simulink model "Model_3"  (R2025b)
settings: Solver=VariableStepAuto  StartTime=0.0  StopTime=10.0  RelTol=1e-3
settings Model: Creator=danielborkovec  LastModifiedBy=danielborkovec

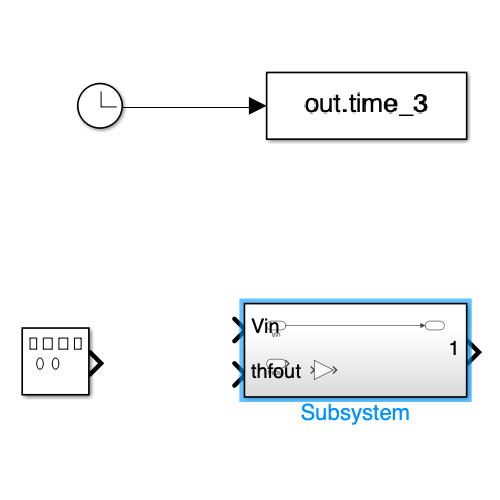
[thumbnail: Simulink's stored preview of the top-level diagram]
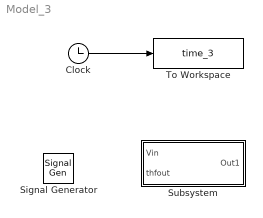
== system Model_3 ==
  Clock : Clock
  Signal Generator : SignalGenerator  Units=rad/sec
  Subsystem : Subsystem
  To Workspace : ToWorkspace  VariableName=time_3  SaveFormat=Timeseries  SampleTime=-1
  wires:
  Clock/1 -> To Workspace/1

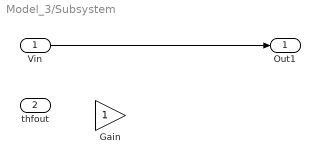
== system Model_3/Subsystem ==
  Vin : Inport
  thfout : Inport  Port=2
  Gain : Gain
  Out1 : Outport
  wires:
  Vin/1 -> Out1/1
